simulink model "Exercise_3"  (R2024a)
settings: Solver=VariableStepAuto  StartTime=0.0  StopTime=100.0  RelTol=1e-3
libraries: fuzblock x1, slpidlib x1
settings Model: Creator=hermangran  LastModifiedBy=hermangran

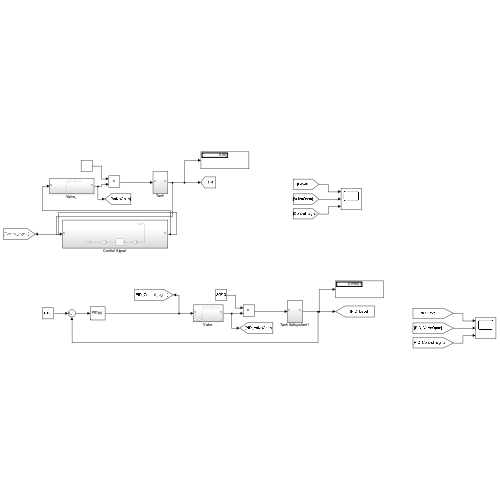
[thumbnail: Simulink's stored preview of the top-level diagram]
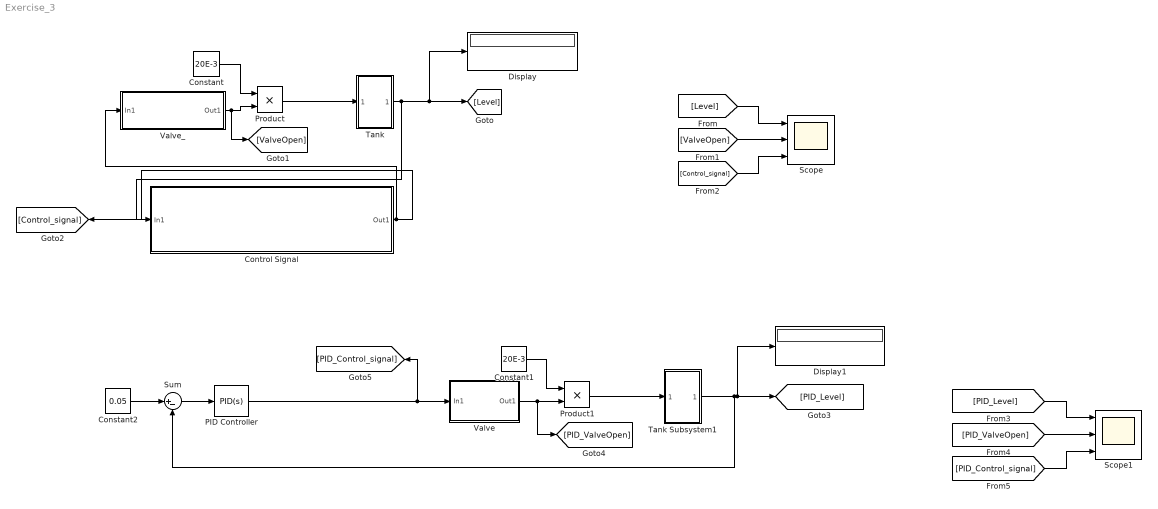
== system Exercise_3 ==
  Constant : Constant  Value=20E-3
  Constant1 : Constant  Value=20E-3
  Constant2 : Constant  Value=0.05
  Control Signal : Subsystem
  Display : Display
      settings: Decimation=3
  Display1 : Display
      settings: Decimation=3
  PID Controller : slpidlib/PID Controller  Controller=PID  Form=Parallel  TimeDomain=Continuous-time  UseExternalTs=off  SampleTime=-1  IntegratorMethod=Forward Euler  FilterMethod=Forward Euler  ControllerParametersSource=internal  P=0  I=1.3262  UseKiTs=off  D=755.7009  UseExternalDerivativeSource=off  N=3  UseFilter=on  TunerSelectOption=Frequency Response Based  InitialConditionSource=internal  InitialConditionForIntegrator=0  InitialConditionForFilter=0  DifferentiatorICPrevScaledInput=0  ExternalReset=none  TrackingMode=off  Kt=1  LimitOutput=off  SatLimitsSource=internal  UpperSaturationLimit=inf  LowerSaturationLimit=-inf  LinearizeAsGain=on  AntiWindupMode=none  Kb=1  LimitIntegrator=off  UpperIntegratorSaturationLimit=inf  LowerIntegratorSaturationLimit=-inf  POutMin=[]  POutMax=[]  IOutMin=[]  IOutMax=[]  DOutMin=[]  DOutMax=[]  NOutMin=[]  NOutMax=[]  SumOutMin=[]  SumOutMax=[]  SaturationOutMin=[]  SaturationOutMax=[]  PParamMin=[]  PParamMax=[]  IParamMin=[]  IParamMax=[]  DParamMin=[]  DParamMax=[]  NParamMin=[]  NParamMax=[]  KbParamMin=[]  KbParamMax=[]  KtParamMin=[]  KtParamMax=[]  KbOutMin=[]  KbOutMax=[]  KtOutMin=[]  KtOutMax=[]  IntegratorOutMin=[]  IntegratorOutMax=[]  FilterOutMin=[]  FilterOutMax=[]  SumI1OutMin=[]  SumI1OutMax=[]  SumI2OutMin=[]  SumI2OutMax=[]  SumI3OutMin=[]  SumI3OutMax=[]  SumI4OutMin=[]  SumI4OutMax=[]  SumDOutMin=[]  SumDOutMax=[]  DifferentiatorOutMin=[]  DifferentiatorOutMax=[]  FilterDiffOutCoefMin=[]  FilterDiffOutCoefMax=[]  ReciprocalOutMin=[]  ReciprocalOutMax=[]  SumDenOutMin=[]  SumDenOutMax=[]  SumNumOutMin=[]  SumNumOutMax=[]  DivideOutMin=[]  DivideOutMax=[]  UdiffTsProdOutMin=[]  UdiffTsProdOutMax=[]  NTsProdOutMin=[]  NTsProdOutMax=[]  UintegralTsProdOutMin=[]  UintegralTsProdOutMax=[]  UngainTsProdOutMin=[]  UngainTsProdOutMax=[]  ClampingZeroOutDataTypeStr=Inherit: Inherit via back propagation  ClampingZeroOutMin=[]  ClampingZeroOutMax=[]  FilterDenConstantOutDataTypeStr=Inherit: Inherit via back propagation  FilterDenConstantOutMin=[]  FilterDenConstantOutMax=[]  PCopyOutDataTypeStr=Inherit: Inherit via back propagation  PCopyOutMin=[]  PCopyOutMax=[]  NCopyOutDataTypeStr=Inherit: Inherit via back propagation  NCopyOutMin=[]  NCopyOutMax=[]  IntegratorContinuousStateAttributes=''  IntegratorStateMustResolveToSignalObject=off  IntegratorRTWStateStorageClass=Auto  FilterContinuousStateAttributes=''  FilterStateMustResolveToSignalObject=off  FilterRTWStateStorageClass=Auto  ParallelPVariant=InternalParameters  IdealPVariant=Disabled  IVariant=InternalParameters  DVariant=InternalParameters  IntegratorVariant=Continuous  SatVariant=Disabled  AWVariant=Passthrough  PCopyVariant=Disabled  TRVariant=Disabled  FdbkBlocksVariant=Forward  IdealPFdbkVariant=Disabled  SatFdbkVariant=Disabled  DerivativeFilterVariant=ContFilter  NVariant=InternalParameters  NCopyVariant=Disabled  FilterICVariant=InternalICsFilter  IntegratorICVariant=InternalICs  ExternalResetVariant=Disabled  TRSumVariant=Passthrough  SumFdbkVariant=Disabled  SumVariant=Sum_PID  TsampFilterVariant=InternalTs  TsampNgainVariant=Passthrough  TsampIntegralVariant=Disabled_SignalSpec  ExternalSaturationOutDataTypeStr=Inherit: Same as second input  DerivativeSourceVariant=ErrorSignal
  Product : Product
  Product1 : Product
  Scope : Scope  NumInputPorts=3
  Scope1 : Scope  NumInputPorts=3
  Sum : Sum  Inputs=|+-
  Tank : Subsystem
  Tank Subsystem1 : Subsystem
  Valve : Subsystem
  Valve_ : Subsystem
  wires:
  Product/1 -> Tank/1(In1)
  Tank/1(Out1) -> [Level], Display/1, Control Signal/1(In1)
  Constant/1 -> Product/1
  [Level] -> Scope/1
  [ValveOpen] -> Scope/2
  [Control_signal] -> Scope/3
  Constant1/1 -> Product1/1
  [PID_Level] -> Scope1/1
  [PID_ValveOpen] -> Scope1/2
  Product1/1 -> Tank Subsystem1/1(In1)
  [PID_Control_signal] -> Scope1/3
  Valve/1(Out1) -> [PID_ValveOpen], Product1/2
  Constant2/1 -> Sum/1
  Tank Subsystem1/1(Out1) -> [PID_Level], Display1/1, Sum/2
  Valve_/1(Out1) -> Product/2, [ValveOpen]
  Control Signal/1(Out1) -> [Control_signal], Valve_/1(In1)
  PID Controller/1 -> [PID_Control_signal], Valve/1(In1)
  Sum/1 -> PID Controller/1

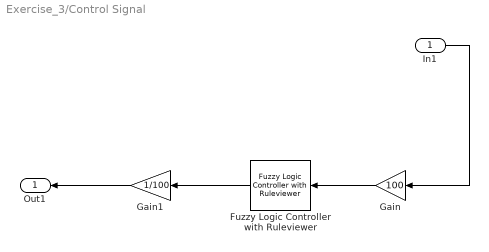
== system Exercise_3/Control Signal ==
  In1 : Inport
  Fuzzy Logic Controller with Ruleviewer : fuzblock/Fuzzy Logic  Controller  with Ruleviewer  fismatrix=levelcontroller  Ts=2
  Gain : Gain  Gain=100
  Gain1 : Gain  Gain=1/100
  Out1 : Outport
  wires:
  Gain1/1 -> Out1/1
  Gain/1 -> Fuzzy Logic Controller with Ruleviewer/1
  In1/1 -> Gain/1
  Fuzzy Logic Controller with Ruleviewer/1 -> Gain1/1

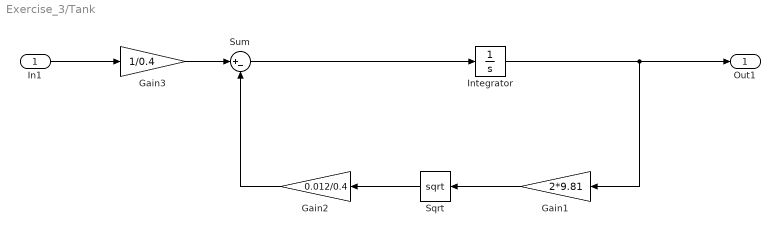
== system Exercise_3/Tank ==
  In1 : Inport
  Gain1 : Gain  Gain=2*9.81
  Gain2 : Gain  Gain=0.012/0.4
  Gain3 : Gain  Gain=1/0.4
  Integrator : Integrator
  Sqrt : Sqrt
  Sum : Sum  Inputs=|+-
  Out1 : Outport
  wires:
  In1/1 -> Gain3/1
  Sqrt/1 -> Gain2/1
  Gain1/1 -> Sqrt/1
  Integrator/1 -> Out1/1, Gain1/1
  Gain3/1 -> Sum/1
  Gain2/1 -> Sum/2
  Sum/1 -> Integrator/1

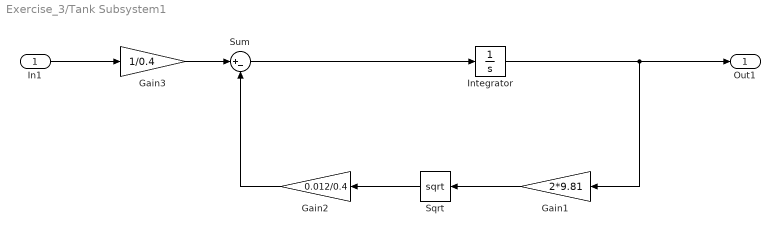
== system Exercise_3/Tank Subsystem1 ==
  In1 : Inport
  Gain1 : Gain  Gain=2*9.81
  Gain2 : Gain  Gain=0.012/0.4
  Gain3 : Gain  Gain=1/0.4
  Integrator : Integrator
  Sqrt : Sqrt
  Sum : Sum  Inputs=|+-
  Out1 : Outport
  wires:
  In1/1 -> Gain3/1
  Sqrt/1 -> Gain2/1
  Gain1/1 -> Sqrt/1
  Integrator/1 -> Out1/1, Gain1/1
  Gain3/1 -> Sum/1
  Gain2/1 -> Sum/2
  Sum/1 -> Integrator/1

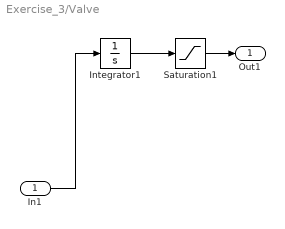
== system Exercise_3/Valve ==
  In1 : Inport
  Integrator1 : Integrator
  Saturation1 : Saturate  UpperLimit=1  LowerLimit=0
  Out1 : Outport
  wires:
  In1/1 -> Integrator1/1
  Saturation1/1 -> Out1/1
  Integrator1/1 -> Saturation1/1

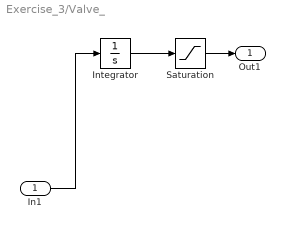
== system Exercise_3/Valve_ ==
  In1 : Inport
  Integrator : Integrator
  Saturation : Saturate  UpperLimit=1  LowerLimit=0
  Out1 : Outport
  wires:
  Saturation/1 -> Out1/1
  In1/1 -> Integrator/1
  Integrator/1 -> Saturation/1
